simulink model "main_sim_acc"  (R2022a)
settings: Solver=ode4  StartTime=t_inicial  StopTime=t_final  FixedStep=t_step  RelTol=1e-3
undefined symbols (not defined in the file): ai, As, Bs, Cs, Ds, L, lambdai, mi, n_max, n_modos, side, tac, v0, v0p, vi, wi, x0
settings Model: VariantFading=off  Creator=LEGION  LastModifiedBy=LEGION

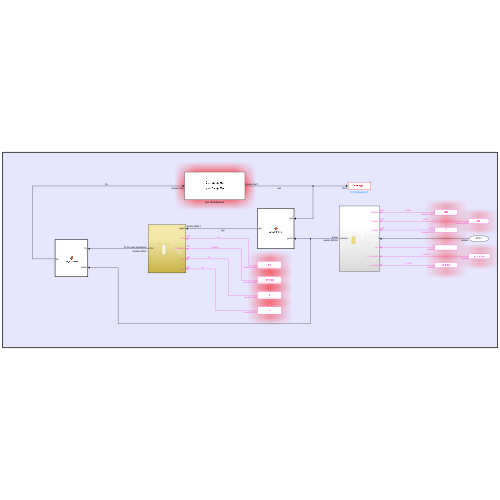
[thumbnail: Simulink's stored preview of the top-level diagram]
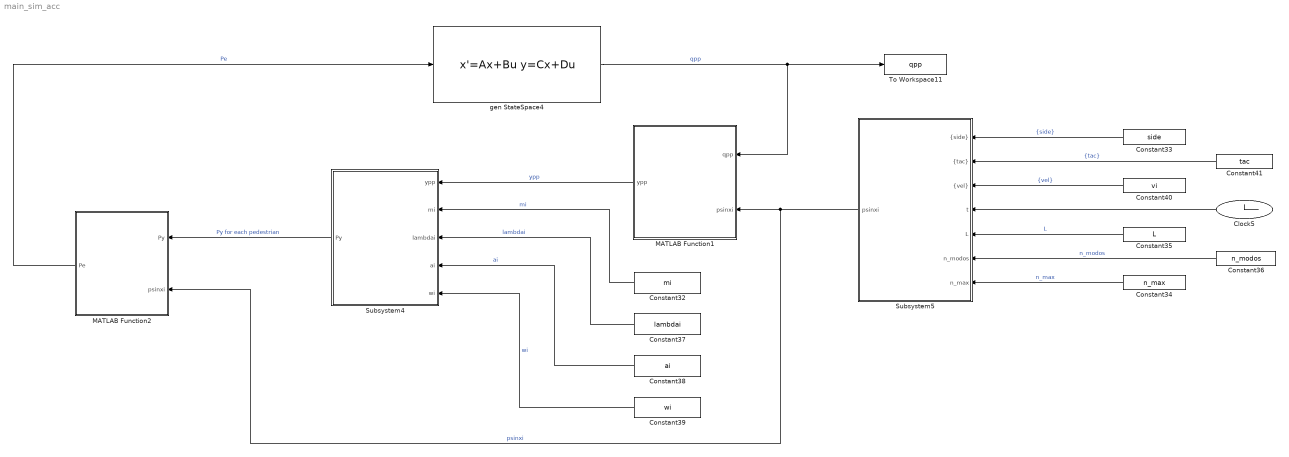
== system main_sim_acc ==
  Clock5 : Clock
  Constant32 : Constant  Value=mi
  Constant33 : Constant  Value=side
  Constant34 : Constant  Value=n_max
  Constant35 : Constant  Value=L
  Constant36 : Constant  Value=n_modos
  Constant37 : Constant  Value=lambdai
  Constant38 : Constant  Value=ai
  Constant39 : Constant  Value=wi
  Constant40 : Constant  Value=vi
  Constant41 : Constant  Value=tac
  MATLAB Function1 : MATLAB Function  TreatAsAtomicUnit=on
  MATLAB Function2 : MATLAB Function  TreatAsAtomicUnit=on
  Subsystem4 : Subsystem
  Subsystem5 : Subsystem
  To Workspace11 : ToWorkspace  VariableName=qpp  SaveFormat=Timeseries  SampleTime=-1
  gen StateSpace4 : StateSpace  A=As  B=Bs  C=Cs  D=Ds  InitialCondition=x0
  wires:
  gen StateSpace4/1 -> MATLAB Function1/1(qpp), To Workspace11/1  "qpp"
  MATLAB Function1/1(ypp) -> Subsystem4/1(ypp)  "ypp"
  Constant38/1 -> Subsystem4/4(ai)  "ai"
  Constant37/1 -> Subsystem4/3(lambdai)  "lambdai"
  Constant32/1 -> Subsystem4/2(mi)  "mi"
  Constant34/1 -> Subsystem5/7(n_max)  "n_max"
  Constant33/1 -> Subsystem5/1("{side}")  "{side}"
  Constant40/1 -> Subsystem5/3("{vel}")  "{vel}"
  Constant36/1 -> Subsystem5/6(n_modos)  "n_modos"
  Constant39/1 -> Subsystem4/5(wi)  "wi"
  Constant41/1 -> Subsystem5/2("{tac}")  "{tac}"
  MATLAB Function2/1(Pe) -> gen StateSpace4/1  "Pe"
  Constant35/1 -> Subsystem5/5(L)  "L"
  Clock5/1 -> Subsystem5/4(t)
  Subsystem4/1(Py) -> MATLAB Function2/1(Py)  "Py for each pedestrian"
  Subsystem5/1(psinxi) -> MATLAB Function1/2(psinxi), MATLAB Function2/2(psinxi)  "psinxi"

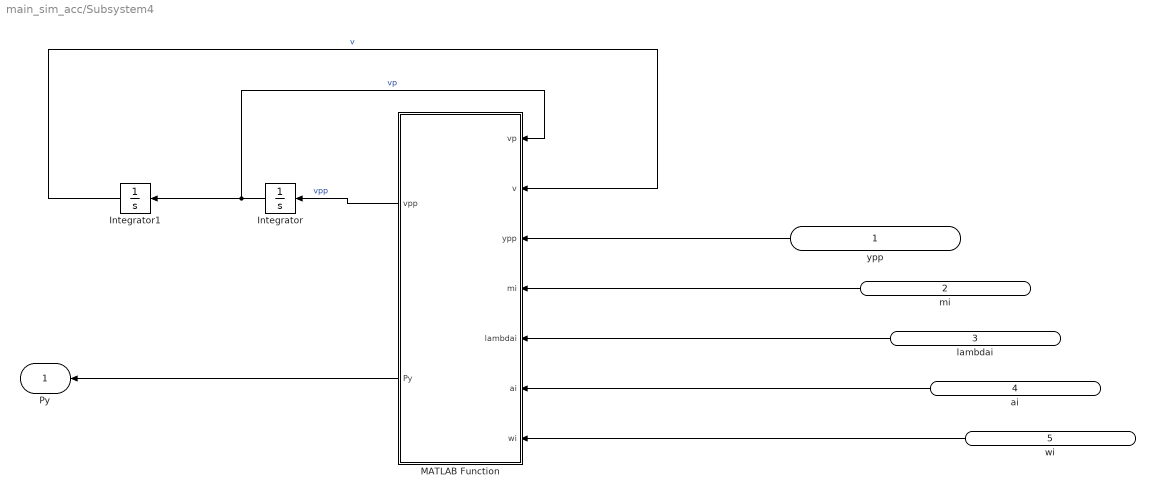
== system main_sim_acc/Subsystem4 ==
  ypp : Inport
  mi : Inport  Port=2
  lambdai : Inport  Port=3
  ai : Inport  Port=4
  wi : Inport  Port=5
  Integrator : Integrator  InitialCondition=v0p
  Integrator1 : Integrator  InitialCondition=v0
  MATLAB Function : MATLAB Function  TreatAsAtomicUnit=on
  Py : Outport
  wires:
  MATLAB Function/1(vpp) -> Integrator/1  "vpp"
  Integrator/1 -> MATLAB Function/1(vp), Integrator1/1  "vp"
  ypp/1 -> MATLAB Function/3(ypp)
  Integrator1/1 -> MATLAB Function/2(v)  "v"
  mi/1 -> MATLAB Function/4(mi)
  lambdai/1 -> MATLAB Function/5(lambdai)
  ai/1 -> MATLAB Function/6(ai)
  wi/1 -> MATLAB Function/7(wi)
  MATLAB Function/2(Py) -> Py/1

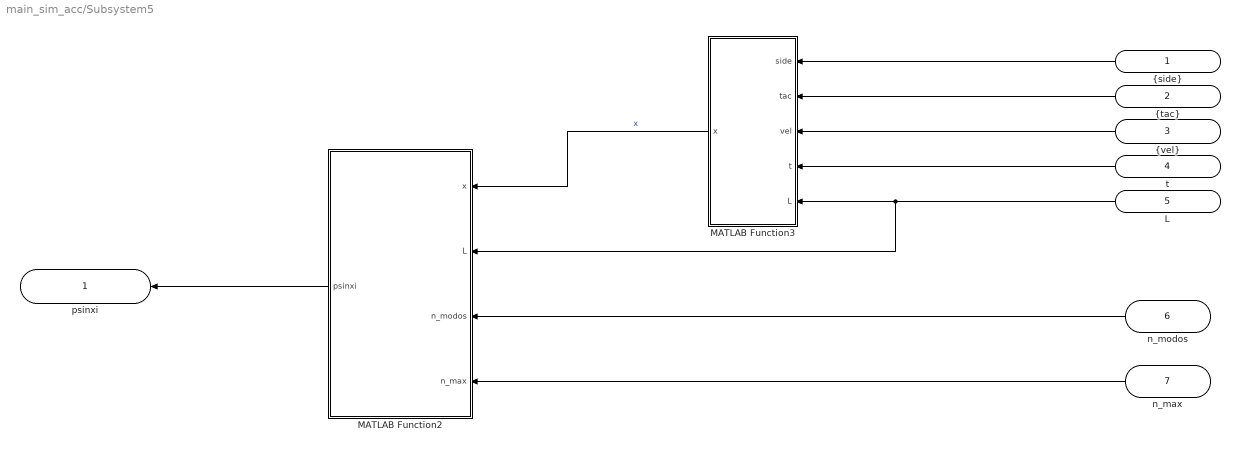
== system main_sim_acc/Subsystem5 ==
  "{side}" : Inport
  "{tac}" : Inport  Port=2
  "{vel}" : Inport  Port=3
  t : Inport  Port=4
  L : Inport  Port=5
  n_modos : Inport  Port=6
  n_max : Inport  Port=7
  MATLAB Function2 : MATLAB Function  TreatAsAtomicUnit=on
  MATLAB Function3 : MATLAB Function  TreatAsAtomicUnit=on
  psinxi : Outport
  wires:
  L/1 -> MATLAB Function3/5(L), MATLAB Function2/2(L)
  MATLAB Function3/1(x) -> MATLAB Function2/1(x)  "x"
  n_modos/1 -> MATLAB Function2/3(n_modos)
  "{side}"/1 -> MATLAB Function3/1(side)
  MATLAB Function2/1(psinxi) -> psinxi/1
  "{tac}"/1 -> MATLAB Function3/2(tac)
  t/1 -> MATLAB Function3/4(t)
  "{vel}"/1 -> MATLAB Function3/3(vel)
  n_max/1 -> MATLAB Function2/4(n_max)

== matlab function main_sim_acc/MATLAB Function1 ==
  data: qpp input; psinxi input; ypp output
function ypp = genToPhys(qpp,psinxi)
% Generar la aceleración que expermentan todos los peatones i (desde el 1
% hasta el peatón p), sumando la respuesta modal de todos los modos (la
% contribución modal)
% ypp = sum(psinxi*qpp,2);                                                    % Sumo todas las contribuciones modales de cada modo
ypp = psinxi*qpp;

== matlab function main_sim_acc/MATLAB Function2 ==
  data: Py input; Pe output; psinxi input
function Pe = physToGen(Py,psinxi)
Pe = psinxi.'*Py;                                                           % Utilicé .' en vez de ' solamente ya que por experiencia me da error a veces si solo ocupo '

== matlab function main_sim_acc/Subsystem4/MATLAB Function ==
  data: vp input; v input; ypp input; vpp output; mi input; lambdai input; ai input; wi input; Py output
function [vpp,Py] = fcn(vp,v,ypp,mi,lambdai,ai,wi)

% Parámetros iniciales
b = 2*pi;
A = 1/(b)^2;
lambda1 = lambdai/(b*(A^2));
lambda2 = lambdai*b/(A^2);
lambda3 = lambdai*b;
% wi = wi/(2*pi)*b; % es igual a wi

% Van Der Pol Type Walker Modificado
fvdv = (lambda1.*(vp.^2) + lambda2.*(v.^2) - lambda3.*ai).*vp + (wi.^2).*v;

% Aceleración del peatón
vpp = -ypp -fvdv;

% Fuerza que aplica el peatón sobre el puente
Py = -mi.*vpp;                                                              % *2 es un factor de escala para que quede acorde al ~10% del peso de la persona, los parámetros de arriba solo ajustan a la forma de vibrar del oscilador

== matlab function main_sim_acc/Subsystem5/MATLAB Function2 ==
  data: x input; psinxi output; L input; n_modos input; n_max input
function psinxi = psinxi(x,L,n_modos,n_max)
    %% Primera forma de hacerlo
% %    psinxi = zeros(n_max,n_modos);
%     
%     % Formar matriz M
%     M = pi/L*ones(n_max,1)*(1:1:n_modos);                                       % Matriz [M]
%     
%     % Formar psinxi
%     psinxi = sin(M.*x);                                                         % [psi_n(x_i)] = sin([M]*{x})
    
    %% Tercera formaforma de hacerlo  (con esta si funciona)
    %Recorriendo cada modo
%     psinxi = zeros(n_max,n_modos);
    psinxi = zeros(200,3);                                                  %%%%%%%%%%% YA SE ME HABÍA OLVIDADO, CUIDADO CON LA CANTIDAD DE PEATONES Y LA CANTIDAD DE MODOS
    for n = 1:n_modos
        psinxi(:,n) = sin(pi*n/L*x);
    end

== matlab function main_sim_acc/Subsystem5/MATLAB Function3 ==
  data: side input; x output; tac input; vel input; t input; L input
function x = posi(side,tac,vel,t,L)
% Determinar la trayectoria del peatón a lo largo del puente en función
% del tiempo

% Cálculos previos
pd = length(side);                                                          % cantidad de peatones
x0 = L*ones(pd,1).*(side-ones(pd,1));                                       % Posición inicial (izquierda o derecha)

% Determinar si entró
delta = max(t - tac, 0);

% Calcular x_ y posición lineal
x_ = x0 + vel.*delta;                                                       % Distancia recorrida desde ese extremo (posición auxiliar
n = floor(x_./L);                                                           % Cantidad de veces que posición auxiliar superó el largo del puente

% Calcular x (trayectoria)
x = (mod(n,2)==0).*(x_ - n.*L)  +  (mod(n,2)==1).*((n+1).*L - x_);          % siEsPar*(función_par) + siEsImpar*(función_impar)
